simulink model "Utkarsh_2005574_W2_P2"  (R2020b)
settings: Solver=ode23  StartTime=0.0  StopTime=10.0  RelTol=1e-3
PostLoadFcn:
  | Utkarsh_2005574_W2_P2plot
  | 
  | be=2;
  | bv=1;
  | Ie=1;
  | Iv=5;
  | muk=1;
  | mus=1.5;
  | R=1;
InitFcn:
  | be=2;
  | bv=1;
  | Ie=1;
  | Iv=5;
  | muk=1;
  | mus=1.5;
  | R=1;
StartFcn:
  | Utkarsh_2005574_W2_P2plot Start
StopFcn:
  | if exist('Utkarsh_2005574_W2_P2_output')
  |    Utkarsh_2005574_W2_P2plot Stop
  | end
CloseFcn:
  | Utkarsh_2005574_W2_P2plot Close
settings Model: DataDictionary=Utkarsh_2005574_W2_P2_DataDicionary.sldd  Creator=home  LastModifiedBy=home

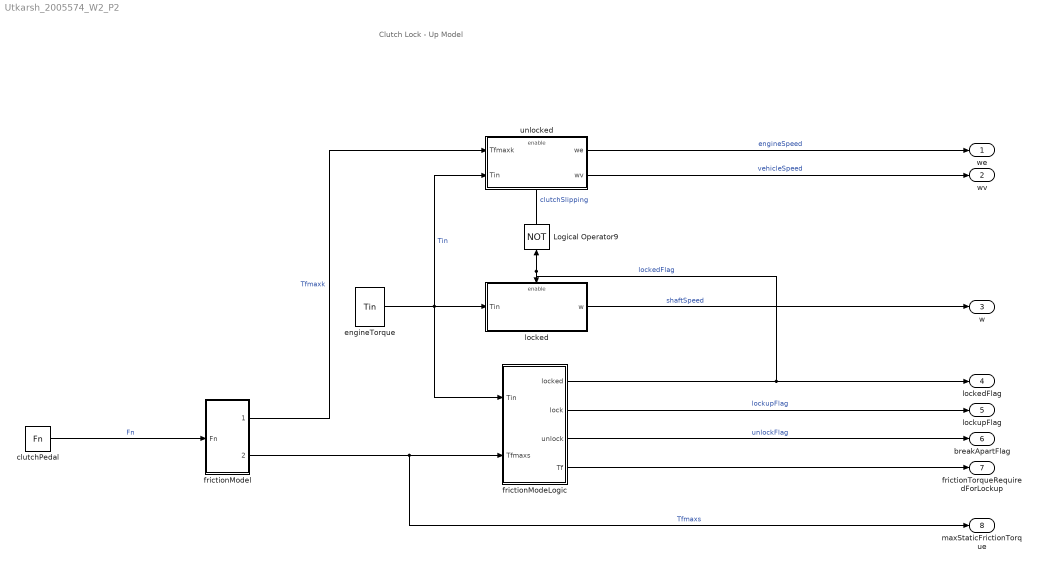
== system Utkarsh_2005574_W2_P2 ==
  note: Clutch Lock - Up Model
  Logical Operator9 : Logic  Operator=NOT  Inputs=1  IconShape=distinctive  OutDataTypeStr=boolean
  clutchPedal : FromWorkspace  VariableName=Fn  ZeroCross=off
  engineTorque : FromWorkspace  VariableName=Tin  ZeroCross=off
  frictionModeLogic : Subsystem
      mask Display: plot([-3 1 1 3 -1 -1],[-1 -1 1 1 1 -1],-4,-5,4,5)
  frictionModel : Subsystem
  locked : Subsystem  TreatAsAtomicUnit=on
      mask Display: plot(-1,-6,6,12,[0 3],[3 3],[3 1 1 3], [1 1 5 5],[2 4 4 2],[4 4 2 2],[4 5],[3 3])
  unlocked : Subsystem  TreatAsAtomicUnit=on
      mask Display: plot(-1,-2,6,8,[0 3],[3 3],[3 1 1 3], [1 1 5 5],[2 4 4 2],[4 4 2 2],[4 5],[3 3])
  we : Outport  InitialOutput=0  VectorParamsAs1DForOutWhenUnconnected=off
  wv : Outport  Port=2  InitialOutput=0  VectorParamsAs1DForOutWhenUnconnected=off
  w : Outport  Port=3  InitialOutput=0  VectorParamsAs1DForOutWhenUnconnected=off
  lockedFlag : Outport  Port=4  InitialOutput=0  VectorParamsAs1DForOutWhenUnconnected=off
  lockupFlag : Outport  Port=5  InitialOutput=0  VectorParamsAs1DForOutWhenUnconnected=off
  breakApartFlag : Outport  Port=6  InitialOutput=0  VectorParamsAs1DForOutWhenUnconnected=off
  frictionTorqueRequiredForLockup : Outport  Port=7  InitialOutput=0  VectorParamsAs1DForOutWhenUnconnected=off
  maxStaticFrictionTorque : Outport  Port=8  InitialOutput=0  VectorParamsAs1DForOutWhenUnconnected=off
  wires:
  frictionModeLogic/4(Tf) -> frictionTorqueRequiredForLockup/1
  locked/1(w) -> w/1  "shaftSpeed"
  unlocked/2(wv) -> wv/1  "vehicleSpeed"
  clutchPedal/1 -> frictionModel/1(Fn)  "Fn"
  frictionModeLogic/1(locked) -> lockedFlag/1, locked/Enable, Logical Operator9/1  "lockedFlag"
  Logical Operator9/1 -> unlocked/Enable  "clutchSlipping"
  frictionModeLogic/3(unlock) -> breakApartFlag/1  "unlockFlag"
  frictionModeLogic/2(lock) -> lockupFlag/1  "lockupFlag"
  frictionModel/2(Tfmaxs) -> frictionModeLogic/2(Tfmaxs), maxStaticFrictionTorque/1  "Tfmaxs"
  unlocked/1(we) -> we/1  "engineSpeed"
  engineTorque/1 -> frictionModeLogic/1(Tin), locked/1(Tin), unlocked/2(Tin)  "Tin"
  frictionModel/1(Tfmaxk) -> unlocked/1(Tfmaxk)  "Tfmaxk"

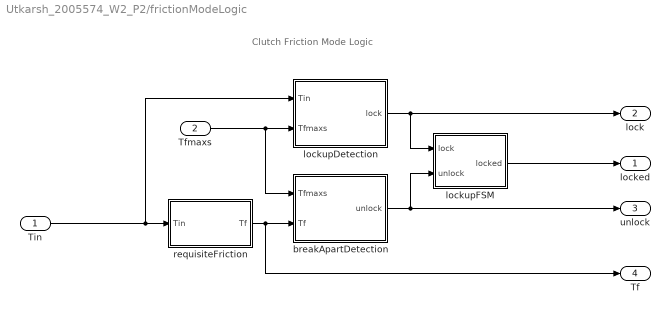
== system Utkarsh_2005574_W2_P2/frictionModeLogic ==
  note: Clutch Friction Mode Logic
  Tin : Inport
  Tfmaxs : Inport  Port=2
  breakApartDetection : Subsystem
  lockupDetection : Subsystem
  lockupFSM : Subsystem
  requisiteFriction : Subsystem
  locked : Outport  InitialOutput=0  VectorParamsAs1DForOutWhenUnconnected=off
  lock : Outport  Port=2  InitialOutput=0  VectorParamsAs1DForOutWhenUnconnected=off
  unlock : Outport  Port=3  InitialOutput=0  VectorParamsAs1DForOutWhenUnconnected=off
  Tf : Outport  Port=4  InitialOutput=0  VectorParamsAs1DForOutWhenUnconnected=off
  wires:
  Tin/1 -> lockupDetection/1(Tin), requisiteFriction/1(Tin)
  Tfmaxs/1 -> lockupDetection/2(Tfmaxs), breakApartDetection/1(Tfmaxs)
  requisiteFriction/1(Tf) -> breakApartDetection/2(Tf), Tf/1
  breakApartDetection/1(unlock) -> lockupFSM/2(unlock), unlock/1
  lockupDetection/1(lock) -> lockupFSM/1(lock), lock/1
  lockupFSM/1(locked) -> locked/1

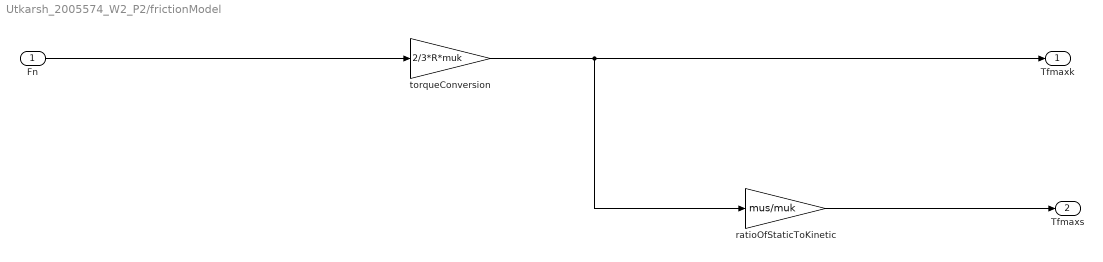
== system Utkarsh_2005574_W2_P2/frictionModel ==
  Fn : Inport
  ratioOfStaticToKinetic : Gain  Gain=mus/muk  SaturateOnIntegerOverflow=on  OutDataTypeStr=Inherit: Same as input  ParamDataTypeStr=Inherit: Same as input
  torqueConversion : Gain  Gain=2/3*R*muk  SaturateOnIntegerOverflow=on  OutDataTypeStr=Inherit: Same as input  ParamDataTypeStr=Inherit: Same as input
  Tfmaxk : Outport  InitialOutput=0  VectorParamsAs1DForOutWhenUnconnected=off
  Tfmaxs : Outport  Port=2  InitialOutput=0  VectorParamsAs1DForOutWhenUnconnected=off
  wires:
  torqueConversion/1 -> Tfmaxk/1, ratioOfStaticToKinetic/1
  Fn/1 -> torqueConversion/1
  ratioOfStaticToKinetic/1 -> Tfmaxs/1

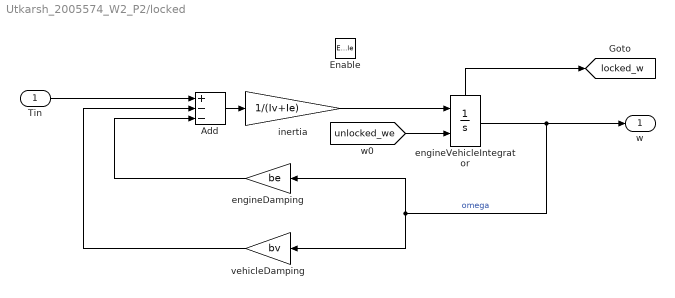
== system Utkarsh_2005574_W2_P2/locked ==
  Tin : Inport
  Enable : EnablePort  StatesWhenEnabling=reset
  Add : Sum  Inputs=+--
  engineDamping : Gain  Gain=be  SaturateOnIntegerOverflow=on  OutDataTypeStr=Inherit: Same as input  ParamDataTypeStr=Inherit: Same as input
  engineVehicleIntegrator : Integrator  InitialConditionSource=external  ShowStatePort=on
  inertia : Gain  Gain=1/(Iv+Ie)  SaturateOnIntegerOverflow=on  OutDataTypeStr=Inherit: Same as input  ParamDataTypeStr=Inherit: Same as input
  vehicleDamping : Gain  Gain=bv  SaturateOnIntegerOverflow=on  OutDataTypeStr=Inherit: Same as input  ParamDataTypeStr=Inherit: Same as input
  w : Outport  InitialOutput=0  VectorParamsAs1DForOutWhenUnconnected=off
  tag scope: locked_w=global
  wires:
  [unlocked_we] -> engineVehicleIntegrator/2
  engineVehicleIntegrator/State -> [locked_w]
  Add/1 -> inertia/1
  Tin/1 -> Add/1
  engineVehicleIntegrator/1 -> w/1, engineDamping/1, vehicleDamping/1  "omega"
  engineDamping/1 -> Add/3
  inertia/1 -> engineVehicleIntegrator/1
  vehicleDamping/1 -> Add/2

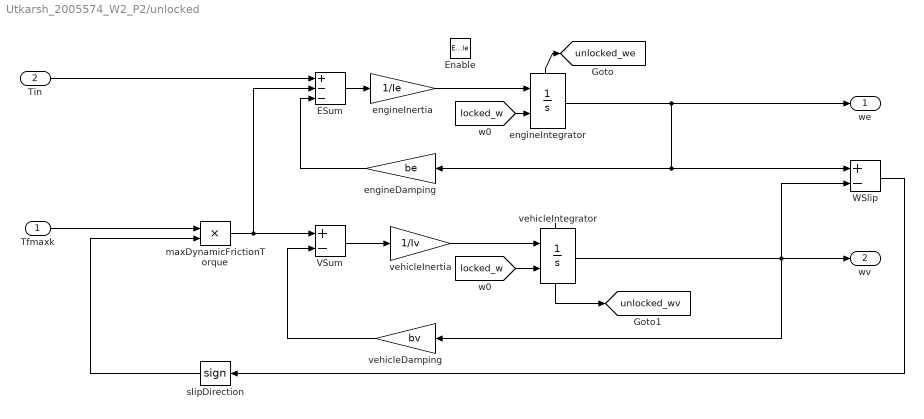
== system Utkarsh_2005574_W2_P2/unlocked ==
  Tfmaxk : Inport
  Tin : Inport  Port=2
  Enable : EnablePort  StatesWhenEnabling=reset
  ESum : Sum  Inputs=+--
  VSum : Sum  Inputs=+-
  WSlip : Sum  Inputs=+-
  engineDamping : Gain  Gain=be  SaturateOnIntegerOverflow=on  OutDataTypeStr=Inherit: Same as input  ParamDataTypeStr=Inherit: Same as input
  engineInertia : Gain  Gain=1/Ie  SaturateOnIntegerOverflow=on  OutDataTypeStr=Inherit: Same as input  ParamDataTypeStr=Inherit: Same as input
  engineIntegrator : Integrator  InitialConditionSource=external  ShowStatePort=on
  maxDynamicFrictionTorque : Product  InputSameDT=on  RndMeth=Zero  SaturateOnIntegerOverflow=on  OutDataTypeStr=Inherit: Same as first input
  slipDirection : Signum
  vehicleDamping : Gain  Gain=bv  SaturateOnIntegerOverflow=on  OutDataTypeStr=Inherit: Same as input  ParamDataTypeStr=Inherit: Same as input
  vehicleInertia : Gain  Gain=1/Iv  SaturateOnIntegerOverflow=on  OutDataTypeStr=Inherit: Same as input  ParamDataTypeStr=Inherit: Same as input
  vehicleIntegrator : Integrator  InitialConditionSource=external  ShowStatePort=on
  we : Outport  InitialOutput=0  VectorParamsAs1DForOutWhenUnconnected=off
  wv : Outport  Port=2  InitialOutput=0  VectorParamsAs1DForOutWhenUnconnected=off
  tag scope: unlocked_we=global, unlocked_wv=global
  wires:
  VSum/1 -> vehicleInertia/1
  vehicleDamping/1 -> VSum/2
  maxDynamicFrictionTorque/1 -> ESum/2, VSum/1
  Tfmaxk/1 -> maxDynamicFrictionTorque/1
  slipDirection/1 -> maxDynamicFrictionTorque/2
  WSlip/1 -> slipDirection/1
  engineIntegrator/State -> [unlocked_we]
  engineInertia/1 -> engineIntegrator/1
  ESum/1 -> engineInertia/1
  engineDamping/1 -> ESum/3
  engineIntegrator/1 -> we/1, engineDamping/1, WSlip/1
  [locked_w] -> engineIntegrator/2
  Tin/1 -> ESum/1
  vehicleIntegrator/State -> [unlocked_wv]
  [locked_w] -> vehicleIntegrator/2
  vehicleInertia/1 -> vehicleIntegrator/1
  vehicleIntegrator/1 -> vehicleDamping/1, WSlip/2, wv/1

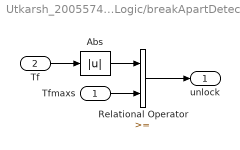
== system Utkarsh_2005574_W2_P2/frictionModeLogic/breakApartDetection ==
  Tfmaxs : Inport
  Tf : Inport  Port=2
  Abs : Abs  SaturateOnIntegerOverflow=on
  Relational Operator : RelationalOperator  OutDataTypeStr=boolean  RndMeth=Nearest  InputSameDT=on
  unlock : Outport  InitialOutput=0  VectorParamsAs1DForOutWhenUnconnected=off
  wires:
  Tf/1 -> Abs/1
  Relational Operator/1 -> unlock/1
  Abs/1 -> Relational Operator/1
  Tfmaxs/1 -> Relational Operator/2

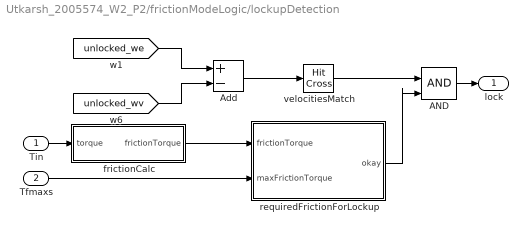
== system Utkarsh_2005574_W2_P2/frictionModeLogic/lockupDetection ==
  Tin : Inport
  Tfmaxs : Inport  Port=2
  AND : Logic  IconShape=distinctive  AllPortsSameDT=off  OutDataTypeStr=boolean
  Add : Sum  Inputs=+-
  frictionCalc : Subsystem
  requiredFrictionForLockup : Subsystem
  velocitiesMatch : HitCross
  lock : Outport  InitialOutput=0  VectorParamsAs1DForOutWhenUnconnected=off
  wires:
  frictionCalc/1(frictionTorque) -> requiredFrictionForLockup/1(frictionTorque)
  Tfmaxs/1 -> requiredFrictionForLockup/2(maxFrictionTorque)
  velocitiesMatch/1 -> AND/1
  AND/1 -> lock/1
  requiredFrictionForLockup/1(okay) -> AND/2
  [unlocked_we] -> Add/1
  [unlocked_wv] -> Add/2
  Add/1 -> velocitiesMatch/1
  Tin/1 -> frictionCalc/1(torque)

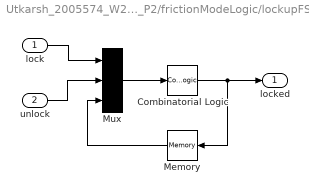
== system Utkarsh_2005574_W2_P2/frictionModeLogic/lockupFSM ==
  lock : Inport
  unlock : Inport  Port=2
  Combinatorial Logic : CombinatorialLogic  TruthTable=[0;1;0;0;1;1;1;0]
  Memory : Memory
  Mux : Mux  Inputs=3
  locked : Outport  InitialOutput=0  VectorParamsAs1DForOutWhenUnconnected=off
  wires:
  Memory/1 -> Mux/3
  Combinatorial Logic/1 -> locked/1, Memory/1
  unlock/1 -> Mux/2
  lock/1 -> Mux/1
  Mux/1 -> Combinatorial Logic/1

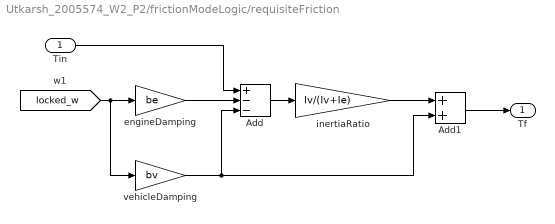
== system Utkarsh_2005574_W2_P2/frictionModeLogic/requisiteFriction ==
  Tin : Inport
  Add : Sum  Inputs=+--
  Add1 : Sum
  engineDamping : Gain  Gain=be  SaturateOnIntegerOverflow=on  OutDataTypeStr=Inherit: Same as input  ParamDataTypeStr=Inherit: Same as input
  inertiaRatio : Gain  Gain=Iv/(Iv+Ie)  SaturateOnIntegerOverflow=on  OutDataTypeStr=Inherit: Same as input  ParamDataTypeStr=Inherit: Same as input
  vehicleDamping : Gain  Gain=bv  SaturateOnIntegerOverflow=on  OutDataTypeStr=Inherit: Same as input  ParamDataTypeStr=Inherit: Same as input
  Tf : Outport  InitialOutput=0  VectorParamsAs1DForOutWhenUnconnected=off
  wires:
  [locked_w] -> vehicleDamping/1, engineDamping/1
  engineDamping/1 -> Add/2
  vehicleDamping/1 -> Add1/2, Add/3
  Add/1 -> inertiaRatio/1
  Tin/1 -> Add/1
  inertiaRatio/1 -> Add1/1
  Add1/1 -> Tf/1

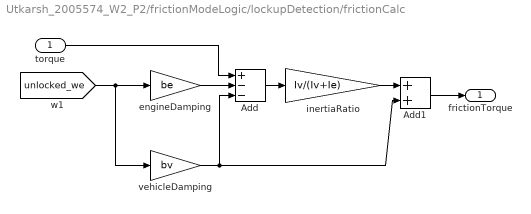
== system Utkarsh_2005574_W2_P2/frictionModeLogic/lockupDetection/frictionCalc ==
  torque : Inport
  Add : Sum  Inputs=+--
  Add1 : Sum
  engineDamping : Gain  Gain=be  SaturateOnIntegerOverflow=on  OutDataTypeStr=Inherit: Same as input  ParamDataTypeStr=Inherit: Same as input
  inertiaRatio : Gain  Gain=Iv/(Iv+Ie)  SaturateOnIntegerOverflow=on  OutDataTypeStr=Inherit: Same as input  ParamDataTypeStr=Inherit: Same as input
  vehicleDamping : Gain  Gain=bv  SaturateOnIntegerOverflow=on  OutDataTypeStr=Inherit: Same as input  ParamDataTypeStr=Inherit: Same as input
  frictionTorque : Outport  InitialOutput=0  VectorParamsAs1DForOutWhenUnconnected=off
  wires:
  [unlocked_we] -> engineDamping/1, vehicleDamping/1
  vehicleDamping/1 -> Add/3, Add1/2
  engineDamping/1 -> Add/2
  Add/1 -> inertiaRatio/1
  inertiaRatio/1 -> Add1/1
  Add1/1 -> frictionTorque/1
  torque/1 -> Add/1

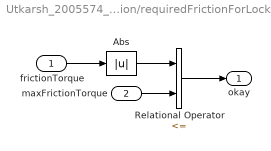
== system Utkarsh_2005574_W2_P2/frictionModeLogic/lockupDetection/requiredFrictionForLockup ==
  frictionTorque : Inport
  maxFrictionTorque : Inport  Port=2
  Abs : Abs  SaturateOnIntegerOverflow=on
  Relational Operator : RelationalOperator  Operator=<=  OutDataTypeStr=boolean  RndMeth=Nearest  InputSameDT=on
  okay : Outport  InitialOutput=0  VectorParamsAs1DForOutWhenUnconnected=off
  wires:
  frictionTorque/1 -> Abs/1
  Relational Operator/1 -> okay/1
  Abs/1 -> Relational Operator/1
  maxFrictionTorque/1 -> Relational Operator/2
